simulink model "test1"  (R2023a)
settings: Solver=FixedStepAuto  StartTime=0.0  StopTime=20  FixedStep=0.01  RelTol=1e-3
libraries: dspnetwork x2, simulink x1
settings Model: Creator=azmol  LastModifiedBy=azmol

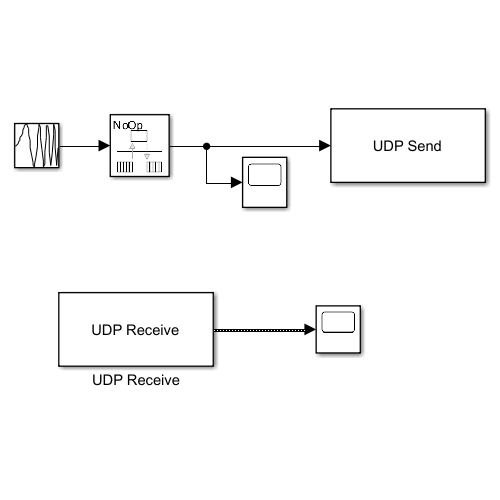
[thumbnail: Simulink's stored preview of the top-level diagram]
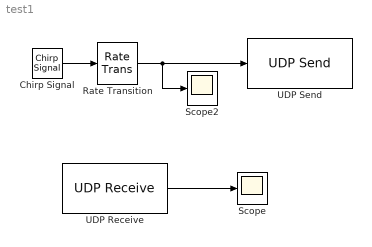
== system test1 ==
  Chirp Signal : simulink/Sources/Chirp Signal  f1=0.1  T=100  f2=1
  Rate Transition : RateTransition
  Scope : Scope
  Scope2 : Scope
  UDP Receive : dspnetwork/UDP Receive  localURL='0.0.0.0'  localPort=25004  remoteURL='192.168.1.7'  remotePort=-1  recvBufferSize=8192  dims=1  signalDatatype=double  isComplex=off  isVarSize=on  showBlockingTime=off  blockingTime=0  sampletime=0.01  blockPlatform=[]
      settings: LibrarySourceBlock=dspsrcs4/UDP Receive
  UDP Send : dspnetwork/UDP Send  remoteURL='127.0.0.1'  remotePort=25000  localURL='0.0.0.0'  localPortSource=Automatically determine  localPort=25001  sendBufferSize=8192  sampletime=-1  blockPlatform=[]  separateLengthPort=0
      settings: LibrarySourceBlock=dspsnks4/UDP Send
  wires:
  UDP Receive/1 -> Scope/1
  Chirp Signal/1 -> Rate Transition/1
  Rate Transition/1 -> UDP Send/1, Scope2/1
